simulink model "OIRT"  (Simulink 8.5)
settings: Solver=ode3  SolverMode=SingleTasking  StartTime=0.0  StopTime=1.0  FixedStep=2e-5  RelTol=1e-4  AbsTol=1e-6
undefined symbols (not defined in the file or in its folder): DAB, den, elements, num
libraries: powerlib x191, powerlib_extras x6
(part 1 of 9)
settings Model: Creator=azadpour  LastModifiedBy=PC  ExtModeTrigMode=oneshot  ExtModeArmWhenConnect=off
settings SolverCC: SolverResetMethod=Robust
settings DataIOCC: LimitDataPoints=off
settings OptimizationCC: BlockReduction=off  BooleanDataType=off  InitFltsAndDblsToZero=on
settings DebuggingCC: SaveWithDisabledLinksMsg=none  SaveWithParameterizedLinksMsg=none  CheckSSInitialOutputMsg=off  SignalResolutionControl=TryResolveAllWithWarning  InheritedTsInSrcMsg=none  DiscreteInheritContinuousMsg=none  MultiTaskDSMMsg=none  MultiTaskCondExecSysMsg=none  TasksWithSamePriorityMsg=none  SigSpecEnsureSampleTimeMsg=none  IntegerOverflowMsg=none  Int32ToFloatConvMsg=none  ParameterPrecisionLossMsg=none  ParameterTunabilityLossMsg=none  FcnCallInpInsideContextMsg=UseLocalSettings  UnconnectedInputMsg=none  UnconnectedOutputMsg=none  UnconnectedLineMsg=none  BusObjectLabelMismatch=none  RootOutportRequireBusObject=none  ModelReferenceDataLoggingMessage=none  StrictBusMsg=None  IntegerSaturationMsg=none
settings HardwareCC: TargetHWDeviceType=32-bit Generic  TargetUnknown=on  ProdEqTarget=off
settings GRTTargetCC: TargetFcnLib=ansi_tfl_tmw.mat

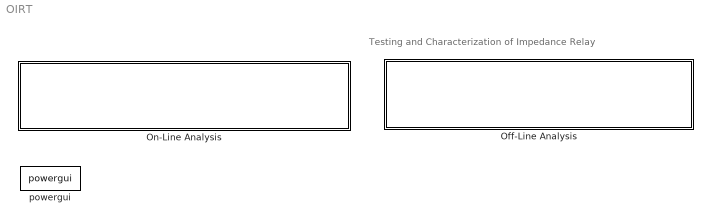
== system OIRT ==
  note: Testing and Characterization of Impedance Relay
  Off-Line Analysis : Subsystem
      mask Display: disp('Off-Line Testing');
  On-Line Analysis : Subsystem  mask(Original Three-phase system with unbalanced source){}
      mask Display: disp('On-Line Testing')
  powergui : powerlib/powergui  SimulationMode=Continuous  SolverType=Tustin/Backward Euler (TBE)  SampleTime=0  frequency=60  SPID=off  DisableSnubberDevices=off  DisableRonSwitches=off  DisableVfSwitches=off  SwTol=0  DisplayEquations=off  Interpol=off  methode=off  Ts=0  FunctionMessages=off  echomessages=off  HookPort=off  EnableUseOfTLC=off  x0status=blocks  frequencyindice=60  Pbase=100e6  ErrMax=1e-4  Iterations=50  UnitsV=kV  UnitsW=MW  buscounter=0  RestoreLinks=warning  ResistiveCurrentMeasurement=off  Frange=[0:2:500]  Ylog=off  Xlog=on  ShowGrid=off  save=off  variable=ZData  structure=0  ZoomFFT=on  StartTime=0.0  cycles=1  DisplayStyle=1  fundamental=60  FreqAxis=off  MaxFrequency=1000  frequencyindicesteady=1  RmsSteady=1  display=off

== system OIRT/Off-Line Analysis ==
  note: Off-Line Impedance Relay Testing
  CB-1 : Subsystem  mask{t_op=0.02}
      mask prompts: t_op "Operating time [s]"
  CB-2 : Subsystem  mask{t_op=0.02}
      mask prompts: t_op "Operating time [s]"
  CB-3 : Subsystem  mask{t_op=0.02}
      mask prompts: t_op "Operating time [s]"
  CT&VT-1 : Subsystem  mask{VT=2000, CT=100}
      mask prompts: VT "VT ratio"; CT "CT ratio"
  CT&VT-2 : Subsystem  mask{VT=2000, CT=100}
      mask prompts: VT "VT ratio"; CT "CT ratio"
  CT&VT-3 : Subsystem  mask{VT=2000, CT=100}
      mask prompts: VT "VT ratio"; CT "CT ratio"
  CurrentP : Scope
      settings: TickLabels=on  YMin=-8000  YMax=9000
  CurrentQ : Scope
      settings: TickLabels=on  YMin=-8000  YMax=9000  SaveName=ScopeData7
  CurrentR : Scope
      settings: TickLabels=on  YMin=-8000  YMax=9000  SaveName=ScopeData16
  Generator P : Subsystem  mask(3-phase inductive source - Ungrounded neutral){V=194367, Phi=10, F=60, R=3.4878, L=0.1323}
      mask prompts: V "Voltage magnitude (V) :"; Phi "Phase angle of phase A (Degrees) :"; F "Frequency (Hz) :"; R "Source resistance (Ohms):"; L "Source inductance (H) :"
      mask init:
      | a=R;b=L;c=inf;
      | short_x =[0,150];
      | short_y =[0,0];
      | 
      | resistor_x = [0 30,30,38,53,68,83,98,113,120,120,150];
      | resistor_y = [0,0,0,25,-25,25,-25,25,-25,0,0,0];
      | 
      | inductor_x = [150,173,173,174,178,184,190,197,202,205,206,204,201,201,197,196,198,201,207,214,220,225,229,229,227,224,224,220,219,221,225,230,237,243,249,252,253,251,247,247,244,243,244,248,254,260,267,272,275,276,276,300];
      | 
      | inductor_y = [0,0,1,11,19,24,25,23,17,8,-2,-12,-18,-18,-9,1,11,19,24,25,23,17,8,-2,-12,-18,-18,-9,1,11,19,24,25,23,17,8,-2,-12,-18,-18,-9,1, 11,19,24,25,23,17,8,0,0,0];
      | 
      | capacitor_x1 = [300 360 360 360];
      | capacitor_y1 = [0 0 25 -25];
      | capacitor_x2 = [390 390 390 450];
      | capacitor_y2 = [25,-25,0,0];
      | if a~=0
      | 	s1=resistor_x;
      | 	s2=resistor_y;
      | else
      | 	s1=short_x;
      | 	s2=short_y;
      | end
      | 
      | if b~=0
      | 	s3=inductor_x;
      | 	s4=inductor_y;
      | else
      | 	s3=short_x+150;
      | 	s4=short_y;
      | end
      | 
      | s5=[];
      | s6=[];
      | s7=[];
      | s8=[];
      mask Display: plot(-170,-60,360,60,s1,s2,s3,s4,s5,s6,s7,s8, [0,9,18,24,29,30,29,24,18,9,0,-9,-18,-24,-29,-30,-29,-24,-18,-9,0]*1.5-45,  [30,29,24,18,9,0,-9,-18,-24,-29,-30,-29,-24,-18,-9,0,9,18,24,29,30]*0.8,[-150,-90],[0,0],[-150,-150],[-20,20],[-165,-165],[-15,15],[-180,-180],[-10,10])
  Generator S : Subsystem  mask(3-phase inductive source - Ungrounded neutral){V=194367, Phi=0, F=60, R=3.4878, L=0.1323}
      mask prompts: V "Voltage magnitude (V) :"; Phi "Phase angle of phase A (Degrees) :"; F "Frequency (Hz) :"; R "Source resistance (Ohms):"; L "Source inductance (H) :"
      mask init: same as OIRT/Off-Line Analysis/Generator P
      mask Display: plot(-170,-60,360,60,s1,s2,s3,s4,s5,s6,s7,s8, [0,9,18,24,29,30,29,24,18,9,0,-9,-18,-24,-29,-30,-29,-24,-18,-9,0]*1.5-45,  [30,29,24,18,9,0,-9,-18,-24,-29,-30,-29,-24,-18,-9,0,9,18,24,29,30]*0.8,[-150,-90],[0,0],[-150,-150],[-20,20],[-165,-165],[-15,15],[-180,-180],[-10,10])
  Line 1 : Subsystem  mask(Teansmission line with fault){ff=60, rr=[0.0815 0.3666], ll=[2.1e-3 6.5e-3], cc=[31.6e-9 12.7e-9], length=40, faultLocation=0.9, faultType='C-A-G', faultR=0.01, faultTime=[9 10 11 12 13]}
      mask prompts: ff "Frequency used for R L C specification (Hz)"; rr "Resistance per unit length (Ohm/mile) [R1 R0]"; ll "Inductance per unit length (H/mile) [L1 L0]"; cc "Capacitance per unit length (F/mile) [C1 C0]"; length "Line length (mile)"; faultLocation "Fault location (p.u.) <0,1>"; faultType "Fault Type"; faultR "Fault Resistance per Phase (Ohm)"; faultTime "Fault time sequence (s) [C O C O C]"
      mask TypeOptions faultType: 'A-G' | 'B-G' | 'C-G' | 'B-C' | 'B-C-G' | 'C-A' | 'C-A-G' | 'A-B-C' | 'A-B-C-G'
  Line 2 : Subsystem  mask(Teansmission line with fault){ff=60, rr=[0.0815 0.3666], ll=[2.1e-3 6.5e-3], cc=[31.6e-9 12.7e-9], length=40, faultLocation=0.6, faultType='A-B-C', faultR=0.01, faultTime=[0.02 10 11 12 13]}
      mask prompts: ff "Frequency used for R L C specification (Hz)"; rr "Resistance per unit length (Ohm/mile) [R1 R0]"; ll "Inductance per unit length (H/mile) [L1 L0]"; cc "Capacitance per unit length (F/mile) [C1 C0]"; length "Line length (mile)"; faultLocation "Fault location (p.u.) <0,1>"; faultType "Fault Type"; faultR "Fault Resistance per Phase (Ohm)"; faultTime "Fault time sequence (s) [C O C O C]"
      mask TypeOptions faultType: 'A-G' | 'B-G' | 'C-G' | 'B-C' | 'B-C-G' | 'C-A' | 'C-A-G' | 'A-B-C' | 'A-B-C-G'
  Line 3 : Subsystem  mask(Teansmission line with fault){ff=60, rr=[0.0815 0.3666], ll=[2.1e-3 6.5e-3], cc=[31.6e-9 12.7e-9], length=40, faultLocation=0.5, faultType='A-G', faultR=0.01, faultTime=[9 10 11 12 13]}
      mask prompts: ff "Frequency used for R L C specification (Hz)"; rr "Resistance per unit length (Ohm/mile) [R1 R0]"; ll "Inductance per unit length (H/mile) [L1 L0]"; cc "Capacitance per unit length (F/mile) [C1 C0]"; length "Line length (mile)"; faultLocation "Fault location (p.u.) <0,1>"; faultType "Fault Type"; faultR "Fault Resistance per Phase (Ohm)"; faultTime "Fault time sequence (s) [C O C O C]"
      mask TypeOptions faultType: 'A-G' | 'B-G' | 'C-G' | 'B-C' | 'B-C-G' | 'C-A' | 'C-A-G' | 'A-B-C' | 'A-B-C-G'
  Mux1 : Mux  Inputs=2
  Mux2 : Mux  Inputs=2
  Mux3 : Mux  Inputs=2
  To File1 : ToFile  Filename=OIRT_VI_Q.mat
  To File2 : ToFile  Filename=OIRT_VI_P.mat
  To File3 : ToFile  Filename=OIRT_VI_R.mat
  VoltageP : Scope
      settings: TickLabels=on  YMin=-8000  YMax=9000  SaveName=ScopeData15
  VoltageQ : Scope
      settings: TickLabels=on  YMin=-8000  YMax=9000  SaveName=ScopeData14
  VoltageR : Scope
      settings: TickLabels=on  YMin=-8000  YMax=9000  SaveName=ScopeData17
  trip : Constant  Value=0
  wires:
  Mux1/1 -> To File2/1
  CT&VT-1/1(Vabcn) -> VoltageP/1, Mux1/1
  CT&VT-1/2(Iabcn) -> Mux1/2, CurrentP/1
  Mux2/1 -> To File1/1
  CT&VT-2/1(Vabcn) -> VoltageQ/1, Mux2/1
  CT&VT-2/2(Iabcn) -> Mux2/2, CurrentQ/1
  Mux3/1 -> To File3/1
  CT&VT-3/1(Vabcn) -> VoltageR/1, Mux3/1
  CT&VT-3/2(Iabcn) -> Mux3/2, CurrentR/1
  trip/1 -> CB-1/1(Trip), CB-2/1(Trip), CB-3/1(Trip)
  connections:
  CB-1/RConn1 -- Line 1/LConn1
  CB-1/RConn2 -- Line 1/LConn2
  CB-1/RConn3 -- Line 1/LConn3
  CB-2/RConn1 -- Line 2/LConn1
  CB-2/RConn2 -- Line 2/LConn2
  CB-2/RConn3 -- Line 2/LConn3
  Line 1/RConn1 -- CT&VT-2/LConn1
  Line 1/RConn2 -- CT&VT-2/LConn2
  Line 1/RConn3 -- CT&VT-2/LConn3
  Line 3/RConn1 -- Generator S/RConn1
  Line 3/RConn2 -- Generator S/RConn2
  Line 3/RConn3 -- Generator S/RConn3
  CB-3/RConn1 -- Line 3/LConn1
  CB-3/RConn2 -- Line 3/LConn2
  CB-3/RConn3 -- Line 3/LConn3
  CT&VT-3/RConn3 -- CB-3/LConn3
  CT&VT-3/RConn2 -- CB-3/LConn2
  CT&VT-3/RConn1 -- CB-3/LConn1
  Line 2/RConn1 -- CT&VT-3/LConn1
  Line 2/RConn2 -- CT&VT-3/LConn2
  Line 2/RConn3 -- CT&VT-3/LConn3
  CT&VT-2/RConn3 -- CB-2/LConn3
  CT&VT-2/RConn2 -- CB-2/LConn2
  CT&VT-2/RConn1 -- CB-2/LConn1
  CT&VT-1/RConn3 -- CB-1/LConn3
  CT&VT-1/RConn2 -- CB-1/LConn2
  CT&VT-1/RConn1 -- CB-1/LConn1
  Generator P/RConn3 -- CT&VT-1/LConn3
  Generator P/RConn2 -- CT&VT-1/LConn2
  Generator P/RConn1 -- CT&VT-1/LConn1

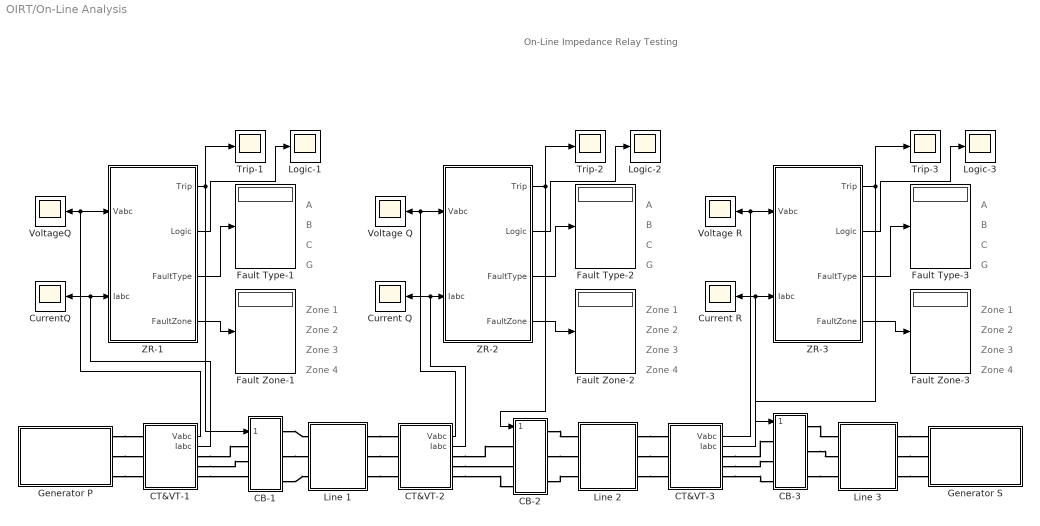
== system OIRT/On-Line Analysis ==
  note: On-Line Impedance Relay Testing
  note: A
  note: B
  note: C
  note: G
  note: Zone 1
  note: Zone 2
  note: Zone 4
  note: Zone 3
  note: A
  note: B
  note: C
  note: G
  note: Zone 1
  note: Zone 2
  note: Zone 4
  note: Zone 3
  note: A
  note: B
  note: C
  note: G
  note: Zone 1
  note: Zone 2
  note: Zone 4
  note: Zone 3
  CB-1 : Subsystem  mask{t_op=0.02}
      mask prompts: t_op "Operating time [s]"
  CB-2 : Subsystem  mask{t_op=0.02}
      mask prompts: t_op "Operating time [s]"
  CB-3 : Subsystem  mask{t_op=0.02}
      mask prompts: t_op "Operating time [s]"
  CT&VT-1 : Subsystem  mask{VT=2000, CT=100}
      mask prompts: VT "VT ratio"; CT "CT ratio"
  CT&VT-2 : Subsystem  mask{VT=2000, CT=100}
      mask prompts: VT "VT ratio"; CT "CT ratio"
  CT&VT-3 : Subsystem  mask{VT=2000, CT=100}
      mask prompts: VT "VT ratio"; CT "CT ratio"
  Current Q : Scope
      settings: TickLabels=on  YMin=-8000  YMax=9000
  Current R : Scope
      settings: TickLabels=on  YMin=-8000  YMax=9000  SaveName=ScopeData5
  CurrentQ : Scope
      settings: TickLabels=on  YMin=-8000  YMax=9000  SaveName=ScopeData10
  Fault Type-1 : Display
  Fault Type-2 : Display
  Fault Type-3 : Display
  Fault Zone-1 : Display
  Fault Zone-2 : Display
  Fault Zone-3 : Display
  Generator P : Subsystem  mask(3-phase inductive source - Ungrounded neutral){V=194367, Phi=10, F=60, R=3.4878, L=0.1323}
      mask prompts: V "Voltage magnitude (V) :"; Phi "Phase angle of phase A (Degrees) :"; F "Frequency (Hz) :"; R "Source resistance (Ohms):"; L "Source inductance (H) :"
      mask init: same as OIRT/Off-Line Analysis/Generator P
      mask Display: plot(-170,-60,360,60,s1,s2,s3,s4,s5,s6,s7,s8, [0,9,18,24,29,30,29,24,18,9,0,-9,-18,-24,-29,-30,-29,-24,-18,-9,0]*1.5-45,  [30,29,24,18,9,0,-9,-18,-24,-29,-30,-29,-24,-18,-9,0,9,18,24,29,30]*0.8,[-150,-90],[0,0],[-150,-150],[-20,20],[-165,-165],[-15,15],[-180,-180],[-10,10])
  Generator S : Subsystem  mask(3-phase inductive source - Ungrounded neutral){V=194367, Phi=0, F=60, R=3.4878, L=0.1323}
      mask prompts: V "Voltage magnitude (V) :"; Phi "Phase angle of phase A (Degrees) :"; F "Frequency (Hz) :"; R "Source resistance (Ohms):"; L "Source inductance (H) :"
      mask init: same as OIRT/Off-Line Analysis/Generator P
      mask Display: plot(-170,-60,360,60,s1,s2,s3,s4,s5,s6,s7,s8, [0,9,18,24,29,30,29,24,18,9,0,-9,-18,-24,-29,-30,-29,-24,-18,-9,0]*1.5-45,  [30,29,24,18,9,0,-9,-18,-24,-29,-30,-29,-24,-18,-9,0,9,18,24,29,30]*0.8,[-150,-90],[0,0],[-150,-150],[-20,20],[-165,-165],[-15,15],[-180,-180],[-10,10])
  Line 1 : Subsystem  mask(Teansmission line with fault){ff=60, rr=[0.0815 0.3666], ll=[2.1e-3 6.5e-3], cc=[31.6e-9 12.7e-9], length=40, faultLocation=0.5, faultType='C-A-G', faultR=0.01, faultTime=[9 10 11 12 13]}
      mask prompts: ff "Frequency used for R L C specification (Hz)"; rr "Resistance per unit length (Ohm/mile) [R1 R0]"; ll "Inductance per unit length (H/mile) [L1 L0]"; cc "Capacitance per unit length (F/mile) [C1 C0]"; length "Line length (mile)"; faultLocation "Fault location (p.u.) <0,1>"; faultType "Fault Type"; faultR "Fault Resistance per Phase (Ohm)"; faultTime "Fault time sequence (s) [C O C O C]"
      mask TypeOptions faultType: 'A-G' | 'B-G' | 'C-G' | 'B-C' | 'B-C-G' | 'C-A' | 'C-A-G' | 'A-B-C' | 'A-B-C-G'
  Line 2 : Subsystem  mask(Teansmission line with fault){ff=60, rr=[0.0815 0.3666], ll=[2.1e-3 6.5e-3], cc=[31.6e-9 12.7e-9], length=40, faultLocation=0.6, faultType='A-B-C', faultR=0.01, faultTime=[0.02 10 11 12 13]}
      mask prompts: ff "Frequency used for R L C specification (Hz)"; rr "Resistance per unit length (Ohm/mile) [R1 R0]"; ll "Inductance per unit length (H/mile) [L1 L0]"; cc "Capacitance per unit length (F/mile) [C1 C0]"; length "Line length (mile)"; faultLocation "Fault location (p.u.) <0,1>"; faultType "Fault Type"; faultR "Fault Resistance per Phase (Ohm)"; faultTime "Fault time sequence (s) [C O C O C]"
      mask TypeOptions faultType: 'A-G' | 'B-G' | 'C-G' | 'B-C' | 'B-C-G' | 'C-A' | 'C-A-G' | 'A-B-C' | 'A-B-C-G'
  Line 3 : Subsystem  mask(Teansmission line with fault){ff=60, rr=[0.0815 0.3666], ll=[2.1e-3 6.5e-3], cc=[31.6e-9 12.7e-9], length=40, faultLocation=0.5, faultType='A-G', faultR=0.01, faultTime=[9 10 11 12 13]}
      mask prompts: ff "Frequency used for R L C specification (Hz)"; rr "Resistance per unit length (Ohm/mile) [R1 R0]"; ll "Inductance per unit length (H/mile) [L1 L0]"; cc "Capacitance per unit length (F/mile) [C1 C0]"; length "Line length (mile)"; faultLocation "Fault location (p.u.) <0,1>"; faultType "Fault Type"; faultR "Fault Resistance per Phase (Ohm)"; faultTime "Fault time sequence (s) [C O C O C]"
      mask TypeOptions faultType: 'A-G' | 'B-G' | 'C-G' | 'B-C' | 'B-C-G' | 'C-A' | 'C-A-G' | 'A-B-C' | 'A-B-C-G'
  Logic-1 : Scope
      settings: SaveName=ScopeData11
  Logic-2 : Scope
      settings: SaveName=ScopeData4
  Logic-3 : Scope
      settings: SaveName=ScopeData6
  Trip-1 : Scope
      settings: TimeRange=0.5  YMin=-0.2  YMax=1.2  SaveName=ScopeData12
  Trip-2 : Scope
      settings: YMin=-0.2  YMax=1.2  SaveName=ScopeData2
  Trip-3 : Scope
      settings: SaveName=ScopeData8
  Voltage Q : Scope
      settings: TickLabels=on  SaveName=ScopeData3
  Voltage R : Scope
      settings: TickLabels=on  SaveName=ScopeData9
  VoltageQ : Scope
      settings: TickLabels=on  SaveName=ScopeData13
  ZR-1 : Subsystem  mask(Distance Relay Settings:){ZoneImpedance=[1.04 2.03 0.52 3.5], ZoneTime=[0 0.33 1 0.66], LineAngle=84.0, k0m1=0.726, k0a1=-3.69, underV=110*0.8}
      mask prompts: ZoneImpedance "Zone impedances [Z1  Z2  Z3  Z4] (Ohm):"; ZoneTime "Zone times [T1  T2  T3  T4] (s):"; LineAngle "Line angle (deg):"; underV "UnderVoltage Threshold (V):"
  ZR-2 : Subsystem  mask(Distance Relay Settings:){ZoneImpedance=[1.04 2.03 0.52 3.5], ZoneTime=[0 0.33 1 0.66], LineAngle=84.0, k0m1=0.726, k0a1=-3.69, underV=110*0.8}
      mask prompts: ZoneImpedance "Zone impedances [Z1  Z2  Z3  Z4] (Ohm):"; ZoneTime "Zone times [T1  T2  T3  T4] (s):"; LineAngle "Line angle (deg):"; underV "UnderVoltage Threshold (V):"
  ZR-3 : Subsystem  mask(Distance Relay Settings:){ZoneImpedance=[1.04 2.03 0.52 3.5], ZoneTime=[0 0.33 1 0.66], LineAngle=84.0, k0m1=0.726, k0a1=-3.69, underV=110*0.8}
      mask prompts: ZoneImpedance "Zone impedances [Z1  Z2  Z3  Z4] (Ohm):"; ZoneTime "Zone times [T1  T2  T3  T4] (s):"; LineAngle "Line angle (deg):"; underV "UnderVoltage Threshold (V):"
  wires:
  ZR-2/3(FaultType) -> Fault Type-2/1
  ZR-2/2(Logic) -> Logic-2/1
  ZR-2/1(Trip) -> Trip-2/1, CB-2/1(Trip)
  ZR-3/4(FaultZone) -> Fault Zone-3/1
  ZR-3/3(FaultType) -> Fault Type-3/1
  ZR-3/2(Logic) -> Logic-3/1
  ZR-3/1(Trip) -> Trip-3/1, CB-3/1(Trip)
  ZR-1/4(FaultZone) -> Fault Zone-1/1
  ZR-1/3(FaultType) -> Fault Type-1/1
  ZR-1/2(Logic) -> Logic-1/1
  CT&VT-1/1(Vabc) -> VoltageQ/1, ZR-1/1(Vabc)
  CT&VT-1/2(Iabc) -> CurrentQ/1, ZR-1/2(Iabc)
  ZR-1/1(Trip) -> Trip-1/1, CB-1/1(Trip)
  CT&VT-2/1(Vabc) -> Voltage Q/1, ZR-2/1(Vabc)
  CT&VT-2/2(Iabc) -> Current Q/1, ZR-2/2(Iabc)
  CT&VT-3/2(Iabc) -> Current R/1, ZR-3/2(Iabc)
  CT&VT-3/1(Vabc) -> Voltage R/1, ZR-3/1(Vabc)
  ZR-2/4(FaultZone) -> Fault Zone-2/1
  connections:
  CB-1/RConn1 -- Line 1/LConn1
  CB-1/RConn2 -- Line 1/LConn2
  CB-1/RConn3 -- Line 1/LConn3
  CB-2/RConn1 -- Line 2/LConn1
  CB-2/RConn2 -- Line 2/LConn2
  CB-2/RConn3 -- Line 2/LConn3
  Line 1/RConn1 -- CT&VT-2/LConn1
  Line 1/RConn2 -- CT&VT-2/LConn2
  Line 1/RConn3 -- CT&VT-2/LConn3
  Line 3/RConn1 -- Generator S/RConn1
  Line 3/RConn2 -- Generator S/RConn2
  Line 3/RConn3 -- Generator S/RConn3
  CB-3/RConn1 -- Line 3/LConn1
  CB-3/RConn2 -- Line 3/LConn2
  CB-3/RConn3 -- Line 3/LConn3
  CT&VT-3/RConn3 -- CB-3/LConn3
  CT&VT-3/RConn2 -- CB-3/LConn2
  CT&VT-3/RConn1 -- CB-3/LConn1
  Line 2/RConn1 -- CT&VT-3/LConn1
  Line 2/RConn2 -- CT&VT-3/LConn2
  Line 2/RConn3 -- CT&VT-3/LConn3
  CT&VT-2/RConn3 -- CB-2/LConn3
  CT&VT-2/RConn2 -- CB-2/LConn2
  CT&VT-2/RConn1 -- CB-2/LConn1
  CT&VT-1/RConn3 -- CB-1/LConn3
  CT&VT-1/RConn2 -- CB-1/LConn2
  CT&VT-1/RConn1 -- CB-1/LConn1
  Generator P/RConn3 -- CT&VT-1/LConn3
  Generator P/RConn2 -- CT&VT-1/LConn2
  Generator P/RConn1 -- CT&VT-1/LConn1

== system OIRT/Off-Line Analysis/CB-1 ==
  Trip : Inport
  BreakerA : powerlib/Elements/Breaker  InitialState=1  SwitchingTimes="[ 1/60  5/60 ]"  External=on  BreakerResistance=0.01  SnubberResistance=1e6  SnubberCapacitance=inf  Measurements=None  MoreParameters=off  NoBreakLoop=off
  BreakerB : powerlib/Elements/Breaker  InitialState=1  SwitchingTimes="[ 1/60  5/60 ]"  External=on  BreakerResistance=0.01  SnubberResistance=1e6  SnubberCapacitance=inf  Measurements=None  MoreParameters=off  NoBreakLoop=off
  BreakerC : powerlib/Elements/Breaker  InitialState=1  SwitchingTimes="[ 1/60  5/60 ]"  External=on  BreakerResistance=0.01  SnubberResistance=1e6  SnubberCapacitance=inf  Measurements=None  MoreParameters=off  NoBreakLoop=off
  NOT : Logic  Operator=NOT  Inputs=1
  Series RLC Branch1 : powerlib/Elements/Series RLC Branch  LConnTagsString=__new0  RConnTagsString=__new0  BranchType=R  Resistance=1e6  Inductance=1.0  SetiL0=off  InitialCurrent=0  Capacitance=1.0  Setx0=off  InitialVoltage=0  Measurements=None
  Series RLC Branch2 : powerlib/Elements/Series RLC Branch  LConnTagsString=__new0  RConnTagsString=__new0  BranchType=R  Resistance=1e6  Inductance=1.0  SetiL0=off  InitialCurrent=0  Capacitance=1.0  Setx0=off  InitialVoltage=0  Measurements=None
  Series RLC Branch3 : powerlib/Elements/Series RLC Branch  LConnTagsString=__new0  RConnTagsString=__new0  BranchType=R  Resistance=1e6  Inductance=1.0  SetiL0=off  InitialCurrent=0  Capacitance=1.0  Setx0=off  InitialVoltage=0  Measurements=None
  Transport Delay : TransportDelay  DelayTime=t_op+0.001  BufferSize=10240
  A1 : PMIOPort  Tag=PMCPort  Port=1  Side=Left
  B1 : PMIOPort  Tag=PMCPort  Port=2  Side=Left
  C1 : PMIOPort  Tag=PMCPort  Port=3  Side=Left
  A2 : PMIOPort  Tag=PMCPort  Port=4  Side=Right
  B2 : PMIOPort  Tag=PMCPort  Port=5  Side=Right
  C2 : PMIOPort  Tag=PMCPort  Port=6  Side=Right
  wires:
  NOT/1 -> BreakerA/1, BreakerB/1, BreakerC/1
  Transport Delay/1 -> NOT/1
  Trip/1 -> Transport Delay/1
  connections:
  A2/RConn1 -- BreakerA/RConn1 -- Series RLC Branch1/RConn1
  B2/RConn1 -- BreakerB/RConn1 -- Series RLC Branch2/RConn1
  C2/RConn1 -- BreakerC/RConn1 -- Series RLC Branch3/RConn1
  A1/RConn1 -- BreakerA/LConn1 -- Series RLC Branch1/LConn1
  B1/RConn1 -- BreakerB/LConn1 -- Series RLC Branch2/LConn1
  C1/RConn1 -- BreakerC/LConn1 -- Series RLC Branch3/LConn1

== system OIRT/Off-Line Analysis/CB-2 ==
  Trip : Inport
  BreakerA : powerlib/Elements/Breaker  InitialState=1  SwitchingTimes="[ 1/60  5/60 ]"  External=on  BreakerResistance=0.01  SnubberResistance=1e6  SnubberCapacitance=inf  Measurements=None  MoreParameters=off  NoBreakLoop=off
  BreakerB : powerlib/Elements/Breaker  InitialState=1  SwitchingTimes="[ 1/60  5/60 ]"  External=on  BreakerResistance=0.01  SnubberResistance=1e6  SnubberCapacitance=inf  Measurements=None  MoreParameters=off  NoBreakLoop=off
  BreakerC : powerlib/Elements/Breaker  InitialState=1  SwitchingTimes="[ 1/60  5/60 ]"  External=on  BreakerResistance=0.01  SnubberResistance=1e6  SnubberCapacitance=inf  Measurements=None  MoreParameters=off  NoBreakLoop=off
  NOT : Logic  Operator=NOT  Inputs=1
  Series RLC Branch1 : powerlib/Elements/Series RLC Branch  LConnTagsString=__new0  RConnTagsString=__new0  BranchType=R  Resistance=1e6  Inductance=1.0  SetiL0=off  InitialCurrent=0  Capacitance=1.0  Setx0=off  InitialVoltage=0  Measurements=None
  Series RLC Branch2 : powerlib/Elements/Series RLC Branch  LConnTagsString=__new0  RConnTagsString=__new0  BranchType=R  Resistance=1e6  Inductance=1.0  SetiL0=off  InitialCurrent=0  Capacitance=1.0  Setx0=off  InitialVoltage=0  Measurements=None
  Series RLC Branch3 : powerlib/Elements/Series RLC Branch  LConnTagsString=__new0  RConnTagsString=__new0  BranchType=R  Resistance=1e6  Inductance=1.0  SetiL0=off  InitialCurrent=0  Capacitance=1.0  Setx0=off  InitialVoltage=0  Measurements=None
  Transport Delay : TransportDelay  DelayTime=t_op+0.001  BufferSize=10240
  A1 : PMIOPort  Tag=PMCPort  Port=1  Side=Left
  B1 : PMIOPort  Tag=PMCPort  Port=2  Side=Left
  C1 : PMIOPort  Tag=PMCPort  Port=3  Side=Left
  A2 : PMIOPort  Tag=PMCPort  Port=4  Side=Right
  B2 : PMIOPort  Tag=PMCPort  Port=5  Side=Right
  C2 : PMIOPort  Tag=PMCPort  Port=6  Side=Right
  wires:
  Trip/1 -> Transport Delay/1
  Transport Delay/1 -> NOT/1
  NOT/1 -> BreakerC/1, BreakerB/1, BreakerA/1
  connections:
  Series RLC Branch3/LConn1 -- BreakerC/LConn1 -- C1/RConn1
  Series RLC Branch2/LConn1 -- BreakerB/LConn1 -- B1/RConn1
  Series RLC Branch1/LConn1 -- BreakerA/LConn1 -- A1/RConn1
  Series RLC Branch3/RConn1 -- BreakerC/RConn1 -- C2/RConn1
  Series RLC Branch2/RConn1 -- BreakerB/RConn1 -- B2/RConn1
  Series RLC Branch1/RConn1 -- BreakerA/RConn1 -- A2/RConn1

== system OIRT/Off-Line Analysis/CB-3 ==
  Trip : Inport
  BreakerA : powerlib/Elements/Breaker  InitialState=1  SwitchingTimes="[ 1/60  5/60 ]"  External=on  BreakerResistance=0.01  SnubberResistance=1e6  SnubberCapacitance=inf  Measurements=None  MoreParameters=off  NoBreakLoop=off
  BreakerB : powerlib/Elements/Breaker  InitialState=1  SwitchingTimes="[ 1/60  5/60 ]"  External=on  BreakerResistance=0.01  SnubberResistance=1e6  SnubberCapacitance=inf  Measurements=None  MoreParameters=off  NoBreakLoop=off
  BreakerC : powerlib/Elements/Breaker  InitialState=1  SwitchingTimes="[ 1/60  5/60 ]"  External=on  BreakerResistance=0.01  SnubberResistance=1e6  SnubberCapacitance=inf  Measurements=None  MoreParameters=off  NoBreakLoop=off
  NOT : Logic  Operator=NOT  Inputs=1
  Series RLC Branch1 : powerlib/Elements/Series RLC Branch  LConnTagsString=__new0  RConnTagsString=__new0  BranchType=R  Resistance=1e6  Inductance=1.0  SetiL0=off  InitialCurrent=0  Capacitance=1.0  Setx0=off  InitialVoltage=0  Measurements=None
  Series RLC Branch2 : powerlib/Elements/Series RLC Branch  LConnTagsString=__new0  RConnTagsString=__new0  BranchType=R  Resistance=1e6  Inductance=1.0  SetiL0=off  InitialCurrent=0  Capacitance=1.0  Setx0=off  InitialVoltage=0  Measurements=None
  Series RLC Branch3 : powerlib/Elements/Series RLC Branch  LConnTagsString=__new0  RConnTagsString=__new0  BranchType=R  Resistance=1e6  Inductance=1.0  SetiL0=off  InitialCurrent=0  Capacitance=1.0  Setx0=off  InitialVoltage=0  Measurements=None
  Transport Delay : TransportDelay  DelayTime=t_op+0.001  BufferSize=10240
  A1 : PMIOPort  Tag=PMCPort  Port=1  Side=Left
  B1 : PMIOPort  Tag=PMCPort  Port=2  Side=Left
  C1 : PMIOPort  Tag=PMCPort  Port=3  Side=Left
  A2 : PMIOPort  Tag=PMCPort  Port=4  Side=Right
  B2 : PMIOPort  Tag=PMCPort  Port=5  Side=Right
  C2 : PMIOPort  Tag=PMCPort  Port=6  Side=Right
  wires:
  NOT/1 -> BreakerA/1, BreakerB/1, BreakerC/1
  Transport Delay/1 -> NOT/1
  Trip/1 -> Transport Delay/1
  connections:
  A2/RConn1 -- BreakerA/RConn1 -- Series RLC Branch1/RConn1
  B2/RConn1 -- BreakerB/RConn1 -- Series RLC Branch2/RConn1
  C2/RConn1 -- BreakerC/RConn1 -- Series RLC Branch3/RConn1
  A1/RConn1 -- BreakerA/LConn1 -- Series RLC Branch1/LConn1
  B1/RConn1 -- BreakerB/LConn1 -- Series RLC Branch2/LConn1
  C1/RConn1 -- BreakerC/LConn1 -- Series RLC Branch3/LConn1

== system OIRT/Off-Line Analysis/CT&VT-1 ==
  Add : Sum  Inputs=+++
  Add1 : Sum  Inputs=+++
  CT-ratio : Gain  Gain=1/CT  SaturateOnIntegerOverflow=on  OutDataTypeStr=Inherit: Same as input  ParamDataTypeStr=Inherit: Same as input
  Ground : powerlib/Elements/Ground  LConnTagsString=a
  IA : powerlib/Measurements/Current Measurement  PhasorSimulation=off  OutputType=Complex  PSBequivalent=0
  IB : powerlib/Measurements/Current Measurement  PhasorSimulation=off  OutputType=Complex  PSBequivalent=0
  IC : powerlib/Measurements/Current Measurement  PhasorSimulation=off  OutputType=Complex  PSBequivalent=0
  Mux : Mux
  Mux1 : Mux
  VA : powerlib/Measurements/Voltage Measurement  PhasorSimulation=off  OutputType=Complex  PSBequivalent=0
  VB : powerlib/Measurements/Voltage Measurement  PhasorSimulation=off  OutputType=Complex  PSBequivalent=0
  VC : powerlib/Measurements/Voltage Measurement  PhasorSimulation=off  OutputType=Complex  PSBequivalent=0
  VT-ratio : Gain  Gain=1/VT  SaturateOnIntegerOverflow=on  OutDataTypeStr=Inherit: Same as input  ParamDataTypeStr=Inherit: Same as input
  A1 : PMIOPort  Tag=PMCPort  Port=1  Side=Left
  B1 : PMIOPort  Tag=PMCPort  Port=2  Side=Left
  C1 : PMIOPort  Tag=PMCPort  Port=3  Side=Left
  A2 : PMIOPort  Tag=PMCPort  Port=4  Side=Right
  B2 : PMIOPort  Tag=PMCPort  Port=5  Side=Right
  C2 : PMIOPort  Tag=PMCPort  Port=6  Side=Right
  Vabcn : Outport  InitialOutput=0
  Iabcn : Outport  Port=2  InitialOutput=0
  wires:
  Mux1/1 -> VT-ratio/1
  VT-ratio/1 -> Vabcn/1
  Mux/1 -> CT-ratio/1
  CT-ratio/1 -> Iabcn/1
  IA/1 -> Mux/1, Add/1
  IB/1 -> Mux/2, Add/2
  IC/1 -> Mux/3, Add/3
  Add/1 -> Mux/4
  VA/1 -> Mux1/1, Add1/1
  VB/1 -> Mux1/2, Add1/2
  VC/1 -> Mux1/3, Add1/3
  Add1/1 -> Mux1/4
  connections:
  VA/LConn2 -- VB/LConn2 -- Ground/LConn1 -- VC/LConn2
  A1/RConn1 -- IA/LConn1 -- VA/LConn1
  B1/RConn1 -- IB/LConn1 -- VB/LConn1
  C1/RConn1 -- IC/LConn1 -- VC/LConn1
  A2/RConn1 -- IA/RConn1
  IB/RConn1 -- B2/RConn1
  IC/RConn1 -- C2/RConn1

== system OIRT/Off-Line Analysis/CT&VT-2 ==
  Add : Sum  Inputs=+++
  Add1 : Sum  Inputs=+++
  CT-ratio : Gain  Gain=1/CT  SaturateOnIntegerOverflow=on  OutDataTypeStr=Inherit: Same as input  ParamDataTypeStr=Inherit: Same as input
  Ground : powerlib/Elements/Ground  LConnTagsString=a
  IA : powerlib/Measurements/Current Measurement  PhasorSimulation=off  OutputType=Complex  PSBequivalent=0
  IB : powerlib/Measurements/Current Measurement  PhasorSimulation=off  OutputType=Complex  PSBequivalent=0
  IC : powerlib/Measurements/Current Measurement  PhasorSimulation=off  OutputType=Complex  PSBequivalent=0
  Mux : Mux
  Mux1 : Mux
  VA : powerlib/Measurements/Voltage Measurement  PhasorSimulation=off  OutputType=Complex  PSBequivalent=0
  VB : powerlib/Measurements/Voltage Measurement  PhasorSimulation=off  OutputType=Complex  PSBequivalent=0
  VC : powerlib/Measurements/Voltage Measurement  PhasorSimulation=off  OutputType=Complex  PSBequivalent=0
  VT-ratio : Gain  Gain=1/VT  SaturateOnIntegerOverflow=on  OutDataTypeStr=Inherit: Same as input  ParamDataTypeStr=Inherit: Same as input
  A1 : PMIOPort  Tag=PMCPort  Port=1  Side=Left
  B1 : PMIOPort  Tag=PMCPort  Port=2  Side=Left
  C1 : PMIOPort  Tag=PMCPort  Port=3  Side=Left
  A2 : PMIOPort  Tag=PMCPort  Port=4  Side=Right
  B2 : PMIOPort  Tag=PMCPort  Port=5  Side=Right
  C2 : PMIOPort  Tag=PMCPort  Port=6  Side=Right
  Vabcn : Outport  InitialOutput=0
  Iabcn : Outport  Port=2  InitialOutput=0
  wires:
  Mux1/1 -> VT-ratio/1
  VT-ratio/1 -> Vabcn/1
  Mux/1 -> CT-ratio/1
  CT-ratio/1 -> Iabcn/1
  IA/1 -> Mux/1, Add/1
  IB/1 -> Mux/2, Add/2
  IC/1 -> Mux/3, Add/3
  Add/1 -> Mux/4
  VA/1 -> Mux1/1, Add1/1
  VB/1 -> Mux1/2, Add1/2
  VC/1 -> Mux1/3, Add1/3
  Add1/1 -> Mux1/4
  connections:
  VA/LConn2 -- VB/LConn2 -- Ground/LConn1 -- VC/LConn2
  A1/RConn1 -- IA/LConn1 -- VA/LConn1
  B1/RConn1 -- IB/LConn1 -- VB/LConn1
  C1/RConn1 -- IC/LConn1 -- VC/LConn1
  A2/RConn1 -- IA/RConn1
  IB/RConn1 -- B2/RConn1
  IC/RConn1 -- C2/RConn1

== system OIRT/Off-Line Analysis/CT&VT-3 ==
  Add : Sum  Inputs=+++
  Add1 : Sum  Inputs=+++
  CT-ratio : Gain  Gain=1/CT  SaturateOnIntegerOverflow=on  OutDataTypeStr=Inherit: Same as input  ParamDataTypeStr=Inherit: Same as input
  Ground : powerlib/Elements/Ground  LConnTagsString=a
  IA : powerlib/Measurements/Current Measurement  PhasorSimulation=off  OutputType=Complex  PSBequivalent=0
  IB : powerlib/Measurements/Current Measurement  PhasorSimulation=off  OutputType=Complex  PSBequivalent=0
  IC : powerlib/Measurements/Current Measurement  PhasorSimulation=off  OutputType=Complex  PSBequivalent=0
  Mux : Mux
  Mux1 : Mux
  VA : powerlib/Measurements/Voltage Measurement  PhasorSimulation=off  OutputType=Complex  PSBequivalent=0
  VB : powerlib/Measurements/Voltage Measurement  PhasorSimulation=off  OutputType=Complex  PSBequivalent=0
  VC : powerlib/Measurements/Voltage Measurement  PhasorSimulation=off  OutputType=Complex  PSBequivalent=0
  VT-ratio : Gain  Gain=1/VT  SaturateOnIntegerOverflow=on  OutDataTypeStr=Inherit: Same as input  ParamDataTypeStr=Inherit: Same as input
  A1 : PMIOPort  Tag=PMCPort  Port=1  Side=Left
  B1 : PMIOPort  Tag=PMCPort  Port=2  Side=Left
  C1 : PMIOPort  Tag=PMCPort  Port=3  Side=Left
  A2 : PMIOPort  Tag=PMCPort  Port=4  Side=Right
  B2 : PMIOPort  Tag=PMCPort  Port=5  Side=Right
  C2 : PMIOPort  Tag=PMCPort  Port=6  Side=Right
  Vabcn : Outport  InitialOutput=0
  Iabcn : Outport  Port=2  InitialOutput=0
  wires:
  Mux1/1 -> VT-ratio/1
  VT-ratio/1 -> Vabcn/1
  Mux/1 -> CT-ratio/1
  CT-ratio/1 -> Iabcn/1
  IA/1 -> Mux/1, Add/1
  IB/1 -> Mux/2, Add/2
  IC/1 -> Mux/3, Add/3
  Add/1 -> Mux/4
  VA/1 -> Mux1/1, Add1/1
  VB/1 -> Mux1/2, Add1/2
  VC/1 -> Mux1/3, Add1/3
  Add1/1 -> Mux1/4
  connections:
  VA/LConn2 -- VB/LConn2 -- Ground/LConn1 -- VC/LConn2
  A1/RConn1 -- IA/LConn1 -- VA/LConn1
  B1/RConn1 -- IB/LConn1 -- VB/LConn1
  C1/RConn1 -- IC/LConn1 -- VC/LConn1
  A2/RConn1 -- IA/RConn1
  IB/RConn1 -- B2/RConn1
  IC/RConn1 -- C2/RConn1

== system OIRT/Off-Line Analysis/Generator P ==
  Ground : powerlib/Elements/Ground  LConnTagsString=a
  RA : powerlib/Elements/Series RLC Branch  LConnTagsString=__new0  RConnTagsString=__new0  BranchType=RL  Resistance=R  Inductance=L  SetiL0=off  InitialCurrent=0  Capacitance=1.0  Setx0=off  InitialVoltage=0  Measurements=None
  RB : powerlib/Elements/Series RLC Branch  LConnTagsString=__new0  RConnTagsString=__new0  BranchType=RL  Resistance=R  Inductance=L  SetiL0=off  InitialCurrent=0  Capacitance=1.0  Setx0=off  InitialVoltage=0  Measurements=None
  RC : powerlib/Elements/Series RLC Branch  LConnTagsString=__new0  RConnTagsString=__new0  BranchType=RL  Resistance=R  Inductance=L  SetiL0=off  InitialCurrent=0  Capacitance=1.0  Setx0=off  InitialVoltage=0  Measurements=None
  VA : powerlib/Electrical Sources/AC Voltage Source  Amplitude=V  Phase=Phi  Frequency=F  SampleTime=0  Measurements=None
  VB : powerlib/Electrical Sources/AC Voltage Source  Amplitude=V  Phase=Phi-120  Frequency=F  SampleTime=0  Measurements=None
  VC : powerlib/Electrical Sources/AC Voltage Source  Amplitude=V  Phase=Phi+120  Frequency=F  SampleTime=0  Measurements=None
  A : PMIOPort  Tag=PMCPort  Port=1  Side=Right
  B : PMIOPort  Tag=PMCPort  Port=2  Side=Right
  C : PMIOPort  Tag=PMCPort  Port=3  Side=Right
  connections:
  VC/LConn1 -- VA/LConn1 -- Ground/LConn1 -- VB/LConn1
  VA/RConn1 -- RA/LConn1
  VB/RConn1 -- RB/LConn1
  VC/RConn1 -- RC/LConn1
  RA/RConn1 -- A/RConn1
  RB/RConn1 -- B/RConn1
  RC/RConn1 -- C/RConn1

== system OIRT/Off-Line Analysis/Generator S ==
  Ground : powerlib/Elements/Ground  LConnTagsString=a
  RA : powerlib/Elements/Series RLC Branch  LConnTagsString=__new0  RConnTagsString=__new0  BranchType=RL  Resistance=R  Inductance=L  SetiL0=off  InitialCurrent=0  Capacitance=1.0  Setx0=off  InitialVoltage=0  Measurements=None
  RB : powerlib/Elements/Series RLC Branch  LConnTagsString=__new0  RConnTagsString=__new0  BranchType=RL  Resistance=R  Inductance=L  SetiL0=off  InitialCurrent=0  Capacitance=1.0  Setx0=off  InitialVoltage=0  Measurements=None
  RC : powerlib/Elements/Series RLC Branch  LConnTagsString=__new0  RConnTagsString=__new0  BranchType=RL  Resistance=R  Inductance=L  SetiL0=off  InitialCurrent=0  Capacitance=1.0  Setx0=off  InitialVoltage=0  Measurements=None
  VA : powerlib/Electrical Sources/AC Voltage Source  Amplitude=V  Phase=Phi  Frequency=F  SampleTime=0  Measurements=Voltage
  VB : powerlib/Electrical Sources/AC Voltage Source  Amplitude=V  Phase=Phi-120  Frequency=F  SampleTime=0  Measurements=Voltage
  VC : powerlib/Electrical Sources/AC Voltage Source  Amplitude=V  Phase=Phi+120  Frequency=F  SampleTime=0  Measurements=None
  A : PMIOPort  Tag=PMCPort  Port=1  Side=Right
  B : PMIOPort  Tag=PMCPort  Port=2  Side=Right
  C : PMIOPort  Tag=PMCPort  Port=3  Side=Right
  connections:
  RC/RConn1 -- C/RConn1
  RB/RConn1 -- B/RConn1
  RA/RConn1 -- A/RConn1
  VC/RConn1 -- RC/LConn1
  VB/RConn1 -- RB/LConn1
  VA/RConn1 -- RA/LConn1
  VB/LConn1 -- Ground/LConn1 -- VA/LConn1 -- VC/LConn1

== system OIRT/Off-Line Analysis/Line 1 ==
  Fault : Subsystem
  Fault Selector : Subsystem
  Line1 : powerlib/Elements/Distributed Parameters Line  Phases=3  Frequency=ff  Resistance=rr  Inductance=ll  Capacitance=cc  Length=length*faultLocation  x1=[0 -5.89694571843166e-010 124738.740593766 -212189.283290793;6.54170619945592e-005 -5.77215720137888e-010 129933.21735066 -209048.808600493;0.000130834123989118 -5.64385825328002e-010 135048.673113462 -205781.197485759;0.000196251185983678 -5.51212690122181e-010 140081.99683476 -202388.437197301;0.000261668247978237 -5.37704325976313e-010 145030.127417076 -198872.591097331;0.000327085309972796 -5.23868948221207e-010 149890.05557452 -195235.797404694]  x2=[0 -1.53789811195489e-009 119722.235957857 -218720.247893427;6.54170619945592e-005 -1.49693264449657e-009 125079.28619522 -215701.48999533;0.000130834123989118 -1.45505679316515e-009 130360.267435471 -212551.549736678;0.000196251185983678 -1.41229602543898e-009 135561.967964193 -209272.342804744;0.000261668247978237 -1.36867634697268e-009 140681.22428282 -205865.863502422;0.000327085309972796 -1.32422428578138e-009 145714.923032571 -202334.183535366]  x3=[0 -1.51573575196636e-011 190.725617402268 -692.392165078942;6.54170619945592e-005 -1.53551126039978e-011 207.741424317679 -687.478488404287;0.000130834123989118 -1.55435292274896e-011 224.630889915616 -682.146710533664;0.000196251185983678 -1.57224928015127e-011 241.383742593573 -676.400074074286;0.000261668247978237 -1.58918944864661e-011 257.989793832405 -670.242073936345;0.000327085309972796 -1.60516312579669e-011 274.438944392644 -663.676455207529]  x4=[0 1.14113808581465e-011 657.53429535822 -1017.12082929099;6.54170619945592e-005 1.16555050421377e-011 682.415686992918 -1000.59730216297;0.000130834123989118 1.18925407416454e-011 706.882056456463 -983.465245552536;0.000196251185983678 1.21223437995635e-011 730.918524129338 -965.735078597862;0.000261668247978237 1.23447744574342e-011 754.510471843773 -947.417584187625;0.000327085309972796 1.25596974404443e-011 777.643551774026 -928.523902403222]  x5=0.000327085309972796  V1=ones(3,3)  V2=ones(3,3)  I1=ones(3,3)  I2=ones(3,3)  nHarmo=1  Measurements=None
  Line2 : powerlib/Elements/Distributed Parameters Line  Phases=3  Frequency=ff  Resistance=rr  Inductance=ll  Capacitance=cc  Length=length*(1-faultLocation)  x1=[0 -1.34902104317558e-009 140604.305195408 -205918.406126863;7.26856244383991e-006 -1.34408180164363e-009 141168.030834224 -205532.351934431;1.45371248876798e-005 -1.33913246793794e-009 141730.696498646 -205144.754481609;2.18056873315197e-005 -1.33417307922109e-009 142292.297963842 -204755.616678714;2.90742497753596e-005 -1.32920367273114e-009 142852.831012971 -204364.941447624;3.63428122191995e-005 -1.32422428578138e-009 143412.291437213 -203972.731721764]  x2=[0 -1.488744855409e-009 140099.965833094 -206492.060343223;7.26856244383991e-006 -1.48496681499984e-009 140665.265281194 -206107.385977783;1.45371248876798e-005 -1.48117762456761e-009 141229.508529966 -205721.164034252;2.18056873315197e-005 -1.47737731256384e-009 141792.691342733 -205333.397412618;2.90742497753596e-005 -1.47356590752355e-009 142354.809490779 -204944.089024465;3.63428122191995e-005 -1.46974343806505e-009 142915.858753383 -204553.241792954]  x3=[0 5.26812744046773e-011 344.64641484829 -662.319085129994;7.26856244383991e-006 5.26283554454036e-011 346.459994489845 -661.372205352862;1.45371248876798e-005 5.25750413208163e-011 348.270972701597 -660.420359595838;2.18056873315197e-005 5.25213324312299e-011 350.079335885633 -659.46355500595;2.90742497753596e-005 5.2467229179923e-011 351.885070463676 -658.501798767464;3.63428122191995e-005 5.24127319731354e-011 353.688162877185 -657.535098101823]  x4=[0 -4.97571440923268e-011 733.388682273641 -942.640440170045;7.26856244383991e-006 -4.96757263570679e-011 735.968933446272 -940.627284174237;1.45371248876798e-005 -4.95939356266087e-011 738.543658521955 -938.607065383619;2.18056873315197e-005 -4.95117725150831e-011 741.112838168108 -936.579798967208;2.90742497753596e-005 -4.94292376394211e-011 743.676453093787 -934.545500146937;3.63428122191995e-005 -4.93463316193441e-011 746.23448404983 -932.504184197545]  x5=3.63428122191995e-005  V1=ones(3,3)  V2=ones(3,3)  I1=ones(3,3)  I2=ones(3,3)  nHarmo=1  Measurements=None
  Timer : powerlib_extras/Control  Blocks/Timer  t=[0 faultTime]  e=[0 1 0 1 0 1]
  A1 : PMIOPort  Tag=PMCPort  Port=1  Side=Left
  B1 : PMIOPort  Tag=PMCPort  Port=2  Side=Left
  C1 : PMIOPort  Tag=PMCPort  Port=3  Side=Left
  A2 : PMIOPort  Tag=PMCPort  Port=4  Side=Right
  B2 : PMIOPort  Tag=PMCPort  Port=5  Side=Right
  C2 : PMIOPort  Tag=PMCPort  Port=6  Side=Right
  wires:
  Timer/1 -> Fault/5(Tfault)
  Fault Selector/4(faultG) -> Fault/4(faultG)
  Fault Selector/3(faultC) -> Fault/3(faultC)
  Fault Selector/2(faultB) -> Fault/2(faultB)
  Fault Selector/1(faultA) -> Fault/1(faultA)
  connections:
  Line2/RConn3 -- C2/RConn1
  Line2/RConn2 -- B2/RConn1
  Line2/RConn1 -- A2/RConn1
  C1/RConn1 -- Line1/LConn3
  B1/RConn1 -- Line1/LConn2
  A1/RConn1 -- Line1/LConn1
  Fault/LConn3 -- Line1/RConn3 -- Line2/LConn3
  Fault/LConn2 -- Line2/LConn2 -- Line1/RConn2
  Fault/LConn1 -- Line2/LConn1 -- Line1/RConn1

== system OIRT/Off-Line Analysis/Line 2 ==
  Fault : Subsystem
  Fault Selector : Subsystem
  Line1 : powerlib/Elements/Distributed Parameters Line  Phases=3  Frequency=ff  Resistance=rr  Inductance=ll  Capacitance=cc  Length=length*faultLocation  x1=[0 -1.62180404320415e-009 127159.070536388 -214700.768110253;4.36113746630395e-005 -1.60097696301396e-009 130671.642719799 -212581.209978021;8.72227493260789e-005 -1.57971713281063e-009 134148.893873359 -210404.190356002;0.000130834123989118 -1.55803029920515e-009 137589.884083178 -208170.297700676;0.000174445498652158 -1.5359223242291e-009 140993.683236835 -205880.135841517;0.000218056873315197 -1.51339918375015e-009 144359.371274791 -203534.323817772]  x2=[0 -1.00926680554999e-009 123597.900549423 -217226.505139843;4.36113746630395e-005 -9.91293544804787e-010 127152.478058157 -215165.152566964;8.72227493260789e-005 -9.73052333736472e-010 130672.685780305 -213045.640055029;0.000130834123989118 -9.54548103012076e-010 134157.572190657 -210868.540516133;0.000174445498652158 -9.35785854393818e-010 137606.195311486 -208634.442428359;0.000218056873315197 -9.16770659387112e-010 141017.622967169 -206343.949676709]  x3=[0 6.78876593468056e-013 309.701215580984 -674.800293423215;4.36113746630395e-005 8.60035659595088e-013 320.75331878901 -669.617493366349;8.72227493260789e-005 1.04096225489238e-012 331.718721184891 -664.253693216574;0.000130834123989118 1.22160747422994e-012 342.594458779674 -658.710342828971;0.000174445498652158 1.40192248853473e-012 353.377591821135 -652.988940591717;0.000218056873315197 1.58185855798939e-012 364.065205588406 -647.091033021065]  x4=[0 -5.68044272303517e-012 595.955987982648 -1026.91848650734;4.36113746630395e-005 -5.82436522604062e-012 612.758353262198 -1016.98196544988;8.72227493260789e-005 -5.9667133815156e-012 629.395087685371 -1006.7705503939;0.000130834123989118 -6.10744871222551e-012 645.861694281125 -996.287001522762;0.000174445498652158 -6.24653317688832e-012 662.153722064604 -985.534152578638;0.000218056873315197 -6.38392918045717e-012 678.266767240248 -974.514910096487]  x5=0.000218056873315197  V1=ones(3,3)  V2=ones(3,3)  I1=ones(3,3)  I2=ones(3,3)  nHarmo=1  Measurements=None
  Line2 : powerlib/Elements/Distributed Parameters Line  Phases=3  Frequency=ff  Resistance=rr  Inductance=ll  Capacitance=cc  Length=length*(1-faultLocation)  x1=[0 -9.79162206797616e-010 128896.939727551 -214124.670424422;2.90742497753596e-005 -9.66913235683931e-010 131236.113664609 -212699.031557986;5.81484995507193e-005 -9.54548103012076e-010 133559.521356166 -211247.839777373;8.72227493260789e-005 -9.42068294285635e-010 135866.883676188 -209771.269423666;0.000116296999101439 -9.29475308784973e-010 138157.923426274 -208269.497886836;0.000145371248876798 -9.16770659387112e-010 140432.365368959 -206742.70558444]  x2=[0 -4.9785950408368e-010 126531.947038187 -215044.13146978;2.90742497753596e-005 -4.88624641093817e-010 128881.340802297 -213644.358909541;5.81484995507193e-005 -4.79331076456715e-010 131215.251215043 -212218.919866819;8.72227493260789e-005 -4.69979926668573e-010 133533.397888631 -210767.985588854;0.000116296999101439 -4.60572315143663e-010 135835.502329064 -209291.730385788;0.000145371248876798 -4.51109372079372e-010 138121.287969606 -207790.331609735]  x3=[0 5.58990784723332e-012 387.111419995282 -662.744806071128;2.90742497753596e-005 5.71877014500766e-012 394.352190932963 -658.462055832675;5.81484995507193e-005 5.8469454098339e-012 401.545585784273 -654.100200276828;8.72227493260789e-005 5.97441824318617e-012 408.690740360034 -649.659763421584;0.000116296999101439 6.10117333092624e-012 415.786796266485 -645.141278725423;0.000145371248876798 6.22719544514331e-012 422.832901008408 -640.545289023217]  x4=[0 -9.29142119823019e-012 559.171428935641 -1020.03783309462;2.90742497753596e-005 -9.3828268010351e-012 570.317979925586 -1013.84775467321;5.81484995507193e-005 -9.47310518400164e-012 581.396014917658 -1007.53587614544;8.72227493260789e-005 -9.56224550140213e-012 592.404203035662 -1001.10295579824;0.000116296999101439 -9.6502370442321e-012 603.341221794563 -994.549766460052;0.000145371248876798 -9.73706924149682e-012 614.205757259364 -987.877095408002]  x5=0.000145371248876798  V1=ones(3,3)  V2=ones(3,3)  I1=ones(3,3)  I2=ones(3,3)  nHarmo=1  Measurements=None
  Timer : powerlib_extras/Control  Blocks/Timer  t=[0 faultTime]  e=[0 1 0 1 0 1]
  A1 : PMIOPort  Tag=PMCPort  Port=1  Side=Left
  B1 : PMIOPort  Tag=PMCPort  Port=2  Side=Left
  C1 : PMIOPort  Tag=PMCPort  Port=3  Side=Left
  A2 : PMIOPort  Tag=PMCPort  Port=4  Side=Right
  B2 : PMIOPort  Tag=PMCPort  Port=5  Side=Right
  C2 : PMIOPort  Tag=PMCPort  Port=6  Side=Right
  wires:
  Timer/1 -> Fault/5(Tfault)
  Fault Selector/4(faultG) -> Fault/4(faultG)
  Fault Selector/3(faultC) -> Fault/3(faultC)
  Fault Selector/2(faultB) -> Fault/2(faultB)
  Fault Selector/1(faultA) -> Fault/1(faultA)
  connections:
  Line2/RConn3 -- C2/RConn1
  Line2/RConn2 -- B2/RConn1
  Line2/RConn1 -- A2/RConn1
  C1/RConn1 -- Line1/LConn3
  B1/RConn1 -- Line1/LConn2
  A1/RConn1 -- Line1/LConn1
  Fault/LConn3 -- Line1/RConn3 -- Line2/LConn3
  Fault/LConn2 -- Line2/LConn2 -- Line1/RConn2
  Fault/LConn1 -- Line2/LConn1 -- Line1/RConn1
